simulink model "untitled"  (R2021a)
settings: Solver=VariableStepAuto  StartTime=0.0  StopTime=10.0  RelTol=1e-3
libraries: hdlBasic x20, xbsIndex_r4 x1
settings Model: Creator=sl186  LastModifiedBy=sl186

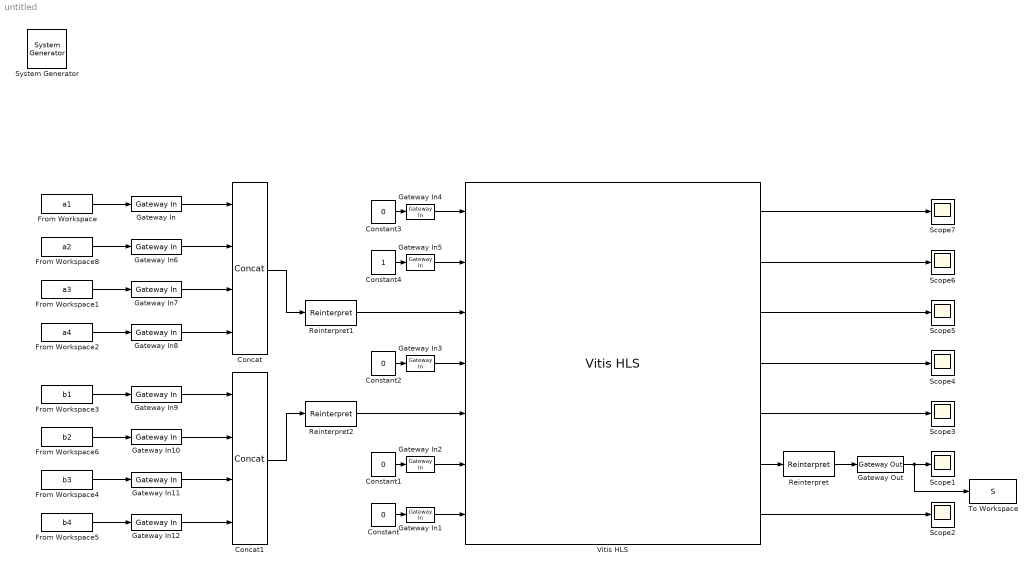
== system untitled ==
  " System Generator" : xbsIndex_r4/ System Generator  Tag=genX  xilinxfamily=kintex7  part=xc7k325t  speed=-3  package=fbg676  synthesis_tool=Vivado  clock_wrapper=Clock Enables  directory=./netlist  proj_type=Vivado  Synth_file=Vivado Synthesis Defaults  Impl_file=Vivado Implementation Defaults  testbench=off  simulink_period=1  sysclk_period=10  dcm_input_clock_period=10  incr_netlist=off  trim_vbits=Everywhere in SubSystem  dbl_ovrd=According to Block Masks  core_generation=According to Block Masks  run_coregen=off  deprecated_control=off  eval_field=0  block_type=sysgen
  Concat : hdlBasic/Concat  num_inputs=4  XmcBlockStatus=1  maskContainerNames=group1  block_type=concat  block_config=sysgen:Concat_config
  Concat1 : hdlBasic/Concat  num_inputs=4  XmcBlockStatus=1  maskContainerNames=group1  block_type=concat  block_config=sysgen:Concat_config
  Constant{,1..3} (4 alike) : Constant  Value=0
  Constant4 : Constant
  From Workspace : FromWorkspace  VariableName=a1
  From Workspace1 : FromWorkspace  VariableName=a3
  From Workspace2 : FromWorkspace  VariableName=a4
  From Workspace3 : FromWorkspace  VariableName=b1
  From Workspace4 : FromWorkspace  VariableName=b3
  From Workspace5 : FromWorkspace  VariableName=b4
  From Workspace6 : FromWorkspace  VariableName=b2
  From Workspace8 : FromWorkspace  VariableName=a2
  Gateway In{,6..12} (8 alike) : hdlBasic/Gateway In  gui_display_data_type=Fixed-point  arith_type=Signed (2's comp)  n_bits=16  bin_pt=10  preci_type=Single  exp_width=8  frac_width=24  rows=1  columns=1  quantization="Round  (unbiased: +/- Inf)"  overflow=Saturate  period=1  UseAsADC=off  ADCChannel='1'  interface=None  automatic_assignment=on  address_offset=hex2dec('00')  intf_name=''  intf_description=''  default_value=0  timing_constraint=None  locs_specified=off  LOCs={}  io_standard={}  inherit_from_input=off  hdl_port=on  XmcBlockStatus=1  maskContainerNames=group4  block_type=gatewayin  block_config=sysgen:gateway_in_config  block_width_w=590  block_height_w=620  block_width=640  block_height=850
  Gateway In{1..5} (5 alike) : hdlBasic/Gateway In  gui_display_data_type=Boolean  arith_type=Boolean  n_bits=16  bin_pt=14  preci_type=Single  exp_width=8  frac_width=24  rows=1  columns=1  quantization="Round  (unbiased: +/- Inf)"  overflow=Saturate  period=1  UseAsADC=off  ADCChannel='1'  interface=None  automatic_assignment=on  address_offset=hex2dec('00')  intf_name=''  intf_description=''  default_value=0  timing_constraint=None  locs_specified=off  LOCs={}  io_standard={}  inherit_from_input=off  hdl_port=on  XmcBlockStatus=1  maskContainerNames=group4  block_type=gatewayin  block_config=sysgen:gateway_in_config  block_width_w=590  block_height_w=620  block_width=640  block_height=850
  Gateway Out : hdlBasic/Gateway Out  inherit_from_input=off  hdl_port=on  rows=1  columns=1  UseAsDAC=off  DACChannel='1'  interface=None  automatic_assignment=on  address_offset=hex2dec('00')  intf_name=''  intf_description=''  timing_constraint=None  locs_specified=off  LOCs={}  io_standard={}  XmcBlockStatus=1  maskContainerNames=group4  block_type=gatewayout  block_config=sysgen:gateway_out_config  block_width_w=590  block_height_w=620  block_width=620  block_height=750
  Reinterpret : hdlBasic/Reinterpret  force_arith_type=on  arith_type="Signed  (2's comp)"  force_bin_pt=on  bin_pt=10  XmcBlockStatus=1  maskContainerNames=group1  block_type=reinterpret  block_config=sysgen:Reinterpret_config
  Reinterpret1 : hdlBasic/Reinterpret  force_arith_type=on  arith_type="Signed  (2's comp)"  force_bin_pt=off  bin_pt=10  XmcBlockStatus=1  maskContainerNames=group1  block_type=reinterpret  block_config=sysgen:Reinterpret_config
  Reinterpret2 : hdlBasic/Reinterpret  force_arith_type=on  arith_type="Signed  (2's comp)"  force_bin_pt=off  bin_pt=10  XmcBlockStatus=1  maskContainerNames=group1  block_type=reinterpret  block_config=sysgen:Reinterpret_config
  Scope{1..7} (7 alike) : Scope
  To Workspace : ToWorkspace  VariableName=S  SaveFormat=Timeseries  SampleTime=-1
  Vitis HLS : hdlBasic/Vitis HLS  anytable='C:\ELEC522\sl186\Assignment3\3_SA_stream\SA_stream\solution1'  fast_sim=off  display_datatype=on  rate_propagation_method=Simulink system period  model_file_path=''  latency=1  block_type=vitis_hls
      settings: infoedit=This block allows including C,C++ and SystemC source files in System Generator for DSP designs.
  wires:
  Vitis HLS/6 -> Reinterpret/1
  Reinterpret1/1 -> Vitis HLS/3
  Concat/1 -> Reinterpret1/1
  Reinterpret/1 -> Gateway Out/1
  Gateway Out/1 -> To Workspace/1, Scope1/1
  Vitis HLS/7 -> Scope2/1
  Vitis HLS/5 -> Scope3/1
  Vitis HLS/1 -> Scope7/1
  Vitis HLS/2 -> Scope6/1
  Vitis HLS/3 -> Scope5/1
  Vitis HLS/4 -> Scope4/1
  Reinterpret2/1 -> Vitis HLS/5
  Concat1/1 -> Reinterpret2/1
  Gateway In1/1 -> Vitis HLS/7
  Constant/1 -> Gateway In1/1
  Gateway In2/1 -> Vitis HLS/6
  Constant1/1 -> Gateway In2/1
  Gateway In3/1 -> Vitis HLS/4
  Constant2/1 -> Gateway In3/1
  Gateway In4/1 -> Vitis HLS/1
  Constant3/1 -> Gateway In4/1
  Gateway In5/1 -> Vitis HLS/2
  Constant4/1 -> Gateway In5/1
  From Workspace/1 -> Gateway In/1
  Gateway In/1 -> Concat/1
  From Workspace8/1 -> Gateway In6/1
  Gateway In6/1 -> Concat/2
  From Workspace2/1 -> Gateway In8/1
  Gateway In8/1 -> Concat/4
  Gateway In7/1 -> Concat/3
  From Workspace1/1 -> Gateway In7/1
  From Workspace6/1 -> Gateway In10/1
  From Workspace4/1 -> Gateway In11/1
  Gateway In10/1 -> Concat1/2
  Gateway In9/1 -> Concat1/1
  From Workspace5/1 -> Gateway In12/1
  From Workspace3/1 -> Gateway In9/1
  Gateway In12/1 -> Concat1/4
  Gateway In11/1 -> Concat1/3
